simulink library "LopesDevelopmentLibrary"  (R2015b)
settings: Solver=ode45  StartTime=0.0  StopTime=10.0  RelTol=1e-3
values from neighbouring files (symbols this model uses):
  d2r = @(d) d*(pi/180)    [LopesDevelopmentLibrary_LoadParameters.m]
  ts = LopesParams.ts    [LopesDevelopmentLibrary_LoadParameters.m]
undefined symbols (not defined in the file or in its folder): anyParameterChanged, DiscIntNeverNeededParam, gcbh, LHF, LKF, LopesParams, macaddr, mxpcnetworkconfig, mxpcrtudprx, mxpcrtudptx, patientParametersChanged, port, PX, PZ, RHF, RKF, SelectorLOPESInSize, StrideTime_s, Time
undefined symbols (not defined in the file): LopesParamsSendDataArrayLen
libraries: LopesDevelopmentLibrary x288, simulink x98, dspmtrx3 x47, xpciplib x6, xpcnetworkbufferlib x5, dspsigops x4, dspstat3 x3, xpcethernetlib x2, visionstatistics x2, xpcseriallib x2, nmc x1, simulink_extras x1
(part 11 of 12)

== matlab function LopesDevelopmentLibrary/Robot control blocks/GeneralLopes/ShowStringInMatlabConsole1 ==
  data pre settings: description=Small string that is put in front of the received text.
  data: stringArray input; len input; pre input; enable input
function fcn(stringArray,len, pre, enable)
%#codegen
persistent t;
if isempty(t)
    t = 0;
end;
t = t+1;
    
coder.extrinsic('fprintf');
if (len~=0 && enable)
    fprintf('%6d: %s  (len = %d) - *%s*\n', t,char(pre'),len,char(stringArray(1:len).')); 
%    feval ('AddToGlobalXX',len);
end;

== matlab function LopesDevelopmentLibrary/Robot control blocks/FromLopes/ShowStringInMatlabConsole ==
  data pre settings: description=Small string that is put in front of the received text.
  data: stringArray input; len input; pre input; enable input
function fcn(stringArray,len, pre, enable)
%#codegen
persistent t;
if isempty(t)
    t = 0;
end;
t = t+1;
    
coder.extrinsic('fprintf');
if (len~=0 && enable)
    fprintf('%6d: %s  (len = %d) - *%s*\n', t,char(pre'),len,char(stringArray(1:len).')); 
%    feval ('AddToGlobalXX',len);
end;

== matlab function LopesDevelopmentLibrary/Robot control blocks/ToLopes/GenerateVelocities/MATLAB Function ==
  data: signalWidth input; forceType input; ena output
function ena = fcn(signalWidth,forceType)
%#codegen
ena=[0,0,0,0]; % We have four outputs
if forceType==-1
    if signalWidth==8
        ena(1)=1;
    else
        ena(2)=1;
    end;
else
    ena(forceType)=1;
end;

== matlab function LopesDevelopmentLibrary/StringFunctions/Pad/pad ==
  data: s input uint8; outArrayLen parameter; y output uint8; y_len output
function [y,y_len]= pad(s,outArrayLen)
%#codegen

% Given s, being an any-(fixed!)-length uint8-array, it outputs
% a 'string' array consisting of a default size (outArrayLen, as a
% parameter),padded with zero's
% together with a length indicating the number of 'valid' bytes in the
% string.
%
% If the string s is too long, it will use the first outputLen-1 chars (and
% add a null-char to fill the whole string up).

y = uint8(zeros(1,outArrayLen));
y_len = min(length(s), outArrayLen-1);
for i=1:y_len,
    y(i) = s(i);
end;

== matlab function LopesDevelopmentLibrary/Robot control blocks/ToLopes/ShowStringInMatlabConsoleIfNotEmpty2 ==
  data pre settings: description=Small string that is put in front of the received text.
  data: stringArray input; len input; pre input; enable input
function fcn(stringArray,len, pre, enable)
%#codegen
persistent t;
if isempty(t)
    t = 0;
end;
t = t+1;
    
coder.extrinsic('fprintf');
if (len~=0 && enable)
    fprintf('%6d: %s  (len = %d) - *%s*\n', t,char(pre'),len,char(stringArray(1:len).')); 
%    feval ('AddToGlobalXX',len);
end;

== matlab function LopesDevelopmentLibrary/StringFunctions/concatWithOptionalDelimiter ==
  data: s1 input; s1_len input; y output uint8; s2 input; s2_len input; y_len output; outputArrayLength parameter
function [y,y_len]= concatWithOptionalDelimiter(s1,s1_len, s2, s2_len, outputArrayLength)
%#codegen

% Concatenates s1 and s2 into y, using a specified delimiter if both strings are non-empty.
%
% s1 and s2 should be uint8-arrays containing a (possibly null-terminated) string.
% Usually, they will be a fixed-length array, holding the string in the
% first part; padded with zeros.
% s1_len and s2_len should be the actual string length (thus, the array
% uint8(['h','o','i',0,0,0,0]) has length 3. Use the strlen block for
% this.
%
% The result of this function is a fixed-length uint8-array, holding the
% string in the first part, padded with zeros, and the length of the
% resulting string (trailing zeros are not counted)
%
% If the resulting string would be too large to fit in the output array,
% it is truncated such that the output array is null-terminated and has
% maximum length.
%
% If s1_len> length(s1) (or similar with s2), the full length of the array
% will be taken as string.
%
% Note on outputArrayLength: The maximum string length is one less because of the trailing null-char

%% Parameters
delimiter = uint8(';'); % Examples: uint8(';'), uint8('; ')
                        % Cannot be a non-empty string (if you don't want a delimiter, remove it from the Add() lines.


%% The work itself

i = 1; % index within y
delimiter_len = length(delimiter);
y=uint8(zeros(outputArrayLength,1));

[y,i] = Add(s1, s1_len,              y, i, outputArrayLength);
if (s1_len~=0 && s2_len ~=0)
    [y,i] = Add(delimiter,delimiter_len, y, i, outputArrayLength);
end;
[y,i] = Add(s2, s2_len,              y, i, outputArrayLength);

y_len = i-1;

%-------------------------------------------------
%% This subfunction actually adds the given string. If the output string
% is alrady 'full', nothing happens.
function [y, i] = Add(whichArray, stringLength, y, i, outputArrayLength)
nToCopy = min([length(whichArray),stringLength, outputArrayLength - i]);
if (nToCopy~=0),
    y(i:(i+nToCopy-1)) = whichArray(1:nToCopy);
    i = i + nToCopy;
end;

== matlab function LopesDevelopmentLibrary/Robot control blocks/ToLopes/ShowStringInMatlabConsoleIfNotEmpty3 ==
  data pre settings: description=Small string that is put in front of the received text.
  data: stringArray input; len input; pre input; enable input
function fcn(stringArray,len, pre, enable)
%#codegen
persistent t;
if isempty(t)
    t = 0;
end;
t = t+1;
    
coder.extrinsic('fprintf');
if (len~=0 && enable)
    fprintf('%6d: %s  (len = %d) - *%s*\n', t,char(pre'),len,char(stringArray(1:len).')); 
%    feval ('AddToGlobalXX',len);
end;

== matlab function LopesDevelopmentLibrary/Robot control blocks/FromLopes/ShowStringInMatlabConsole1 ==
  data pre settings: description=Small string that is put in front of the received text.
  data: stringArray input; len input; pre input; enable input
function fcn(stringArray,len, pre, enable)
%#codegen
persistent t;
if isempty(t)
    t = 0;
end;
t = t+1;
    
coder.extrinsic('fprintf');
if (len~=0 && enable)
    fprintf('%6d: %s  (len = %d) - *%s*\n', t,char(pre'),len,char(stringArray(1:len).')); 
%    feval ('AddToGlobalXX',len);
end;

== matlab function LopesDevelopmentLibrary/StringFunctions/ShowStringInMatlabConsoleIfNotEmpty ==
  data pre settings: description=Small string that is put in front of the received text.
  data: stringArray input; len input; pre input; enable input
function fcn(stringArray,len, pre, enable)
%#codegen
persistent t;
if isempty(t)
    t = 0;
end;
t = t+1;
    
coder.extrinsic('fprintf');
if (len~=0 && enable)
    fprintf('%6d: %s  (len = %d) - *%s*\n', t,char(pre'),len,char(stringArray(1:len).')); 
%    feval ('AddToGlobalXX',len);
end;

== matlab function LopesDevelopmentLibrary/Robot control blocks/ToLopes/makeCreateBiasForceSpring ==
  data: normalBool input; bool output boolean; forceBool input double
function bool  = makeBool(normalBool, forceBool)
%#codegen

% Passes normalBool if forceBool is -1; otherwise it forces the output
% to be equal to forceBool. In diagram:
%
% forceBool | normalBool || Output
% --------------------------------
%     -1    |   false    || false
%     -1    |   true     || true
%      0    |  dont'care || false
% otherwise |  dont'care || true

if forceBool==-1
    bool = normalBool;
elseif forceBool == 0
    bool = false;
else
    bool = true;
end;

== matlab function LopesDevelopmentLibrary/BlocksForInternalUse/GaitGeneration/OrderKeyEvents/SortKeyEvents ==
  data: kE input; kE_out output; Error output double; jointNumber input double
function [kE_out, Error]= fcn(kE, jointNumber)
%#codegen
%
% This function does two things:
% (0.) It does keyEventPhases mod 100 (so that they're in the range [0,100).
% 1. It checks whether the key events (after wrapping around 100) are
%    strictly increasing. If not, it generates an Exception.
%    Note that it is allowed that the key event with the lowest phase
%    is somewhere in the middle, e.g. [50, 66, 95, 101, 7, 20]' as the
%    first column is valid.
% 2. It sorts the key events such that they are strictly increasing (if
%    there are two key events at the same place, the 'first' is decreased a
%    tiny little bit (1e-10) in order to make sure they are strictly
%    increasing again. This whole step is always done, even if an exception
%    was generated.
%
% The underlying reasons:
% 1. If the key events are not in the right order, this is most probably not
%    what we want, so we should stop the whole thing.
% 2. The blocks further on in the data path require a strictly incrasing
%    key event matrix. In order to guarantee that these blocks don't crash,
%    we will make sure that they get what they want, even if the resulting
%    data would not be what we want. The exception can be used to detect
%    this situation, and at least the application does not crash.
%
% Example:
%      [  50   101   102   103 ]
%      [  66   201   202   203 ] 
%      [  95   301   302   303 ]
%  In: [ 101   401   402   403 ]
%      [   7   501   502   503 ]
%      [  20   601   602   603 ]
%  

% Get phase data and wrap them
firstColumn = mod(kE(:,1),100);
kE (:,1) = firstColumn;

% Strict increasingness can be checked by getting the diff of the phase
% data; there should be only one value <=0
nNonPositives = sum(diff([firstColumn;firstColumn(1)]) <=0);

% Exception handling
if (nNonPositives~=1),
    % Then the key events are not in correct order
    Error=jointNumber;
else
    % No error
    Error=0;
end;

while true
    % Sort them (no guarantee on identicity of two adjacent key events
    kE = sortrows(kE,1);

    % Check if we have multiple key events at one spot
    firstColumn = kE(:,1);
    d = diff(firstColumn);
    if (all(d~=0)), break; end; % Then there are no overlaps
    firstColumn(d==0) = mod(firstColumn(d==0)-1,100);
    kE(:,1) = firstColumn;
end;

kE_out = kE;

== matlab function LopesDevelopmentLibrary/BlocksForInternalUse/GaitGeneration/keyEvents2breakscoefs3/keyEvents2breakscoefs3 ==
  data: keyEvents input; breaks output; coefs output
function [breaks,coefs] = keyEvents2breakscoefs3(keyEvents)
%#codegen
%
% Given key-events with x, position and velocity, this function creates
% breaks/coefs for a 3rd order spline

% This function generates a list of breaks and coefs, given a list
% of keyEvents. The keyEvents matrix should have one row for each 'event',
% being [time, position, rate].
% Units:
% - phase [%]
% - position [deg, cm, ...]
% - rate [deg/%, cm/%, ...]
%
% The values in phase should be strictly increasing and 0<=phase<100.
% This function automatically wraps the events, so there is no need to put
% an event at 0.

% Add a key event before zero and one after 100:
kE = [ ...
    keyEvents(end,:) - [100,0,0];
    keyEvents;
    keyEvents(1,:) + [100,0,0]];

% Special case: it may be the case that the user gave a key event at exactly 0 AND
% at exactly 100. In that case, we get repeated key events at 0 and 100
% (because of the previous operation), which is invalid for ppval. We can
% not throw the extra points away because the length of the array is fixed.
% However, we can move them away freely because we will never use the parts
% below 0 and above 100 (and the part between 0 and 100 is not affected).
% Note however that this may give a jump in the position (or velocity)
% of the signal. Therefore, this actually should never happen (with the
% exception of the time signal).
if (kE(1,1) == 0 && kE(2,1) == 0)
    kE(1,1) = -100;
    kE(end,1) = 200;
end;
% For the generation of piecewise polynomials, we need the endpoint data
% of two breaks in one line, so build a matrix:
kE2 = [kE(1:end-1,2:3), kE(2:end,2:3)];

breaks = kE(:,1);
diffbreaks = diff(breaks);
coefs=zeros(size(kE2,1),4); 
for i=1:size(kE2,1),
    % x1 = 0;
    x2 = diffbreaks(i);

    % In theory:
    %   A = [  x1^3,   x1^2,   x1,   1; 
    %        3*x1^2, 2*x1  ,    1,   0;
    %          x2^3,   x2^2,   x2,   1;
    %        3*x2^2, 2*x2  ,    1,   0];
    % However, x1=0, so it becomes:
    A = [0, 0, 0, 1; 0, 0, 1,0; x2^3, x2^2, x2, 1; 3*x2^2, 2*x2, 1,0]; 
    coefs(i,:) = (A \ (kE2(i,:))')';
end;

% pp = mkpp(breaks,coefs);

== matlab function LopesDevelopmentLibrary/StringFunctions/concatDelimiter ==
  data: s1 input; s1_len input; y output; s2 input; s2_len input; y_len output
function [y,y_len]= concatDelimiter(s1,s1_len, s2, s2_len)
%#codegen

% Concatenates s1 and s2 into y, using a ';' as a delimiter.
%
% s1 and s2 should be uint8-arrays containing a (possibly null-terminated) string.
% Usually, they will be a fixed-length array, holding the string in the
% first part; padded with zeros.
% s1_len and s2_len should be the actual string length (thus, the array
% uint8(['h','o','i',0,0,0,0]) has length 3. Use the strlen block for
% this.
%
% The result of this function is a fixed-length uint8-array, holding the
% string in the first part, padded with zeros, and the length of the
% resulting string (trailing zeros are not counted)
%
% If the resulting string would be too large to fit in the output array,
% it is truncated such that the output array is null-terminated and has
% maximum length.
%
% If s1_len> length(s1) (or similar with s2), the full length of the array
% will be taken as string.

%% Parameters
outputArrayLength = uint32(100); % The maximum string length is one less because of the trailing null-char
delimiter = uint8(';'); % Examples: uint8(';'), uint8('; ')
                        % Cannot be a non-empty string (if you don't want a delimiter, remove it from the Add() lines.
delimiter_len = 1;


%% The work itself
i = uint32(1); % index within y
y=zeros(outputArrayLength,1);

[y,i] = Add(s1, s1_len,              y, i, outputArrayLength);
[y,i] = Add(delimiter,delimiter_len, y, i, outputArrayLength);
[y,i] = Add(s2, s2_len,              y, i, outputArrayLength);

y_len = i-1;

%-------------------------------------------------
%% This subfunction actually adds the given string. If the output string
% is alrady 'full', nothing happens.
function [y, i] = Add(whichArray, stringLength, y, i, outputArrayLength)
nToCopy = min([length(whichArray),stringLength, outputArrayLength - i]);
if (nToCopy~=0),
    y(i:(i+nToCopy-1)) = whichArray(1:nToCopy);
    i = i + nToCopy;
end;

== matlab function LopesDevelopmentLibrary/StringFunctions/strlen_as_double ==
  data: s input; len output
function len = strlen(s)
%#codegen

% This function returns the length of the actual string, WITHOUT any
% trailing '\0's. So, the array  ['h','e','l','l','o',0,0,0,0] returns 5.0.
% The output of this function is a double.
%
% s should be a uint8-array containing a string terminated with at least
% one '\0' character. The ASCII Encode block generates such an array
% (the array generated is fixed length, the first n bytes are the string,
% all other bytes are '\0'). 
%
% If the string does not have a trailing '\0' (in other words, if it is
% too large for its containing array), it returns the length of the array.

len = 1.0;
maxlen = length(s);

while (len<= maxlen && s(len)~=0), 
    len = len + 1; 
end;
% Now len is the index of the first trailing '\0' (or maxlen+1);
% that is one more than the string length, so decrease by one:
len = len - 1;

== matlab function LopesDevelopmentLibrary/BlocksForInternalUse/GaitGeneration/keyEvents2breakscoefs5/keyEvents2breakscoefs5 ==
  data: keyEvents input; breaks output; coefs output
function [breaks,coefs] = keyEvents2breakscoefs5(keyEvents)
%#codegen
%
% Given key-events with x, position, velocity and acceleration, this
% function creates breaks/coefs for a 5rd order spline

% This function generates a list of breaks and coefs, given a list
% of keyEvents. The keyEvents matrix should have one row for each 'event',
% being [time, position, rate, rate^2].
% Units:
% - phase [%]
% - position [rad, m, ...]
% - rate [rad/%, m/%, ...]
% - rate^2 [ rad/%^2, m/%^2, ...]
%
% The values in phase should be strictly increasing and 0<=phase<100.
% This function automatically wraps the events, so there is no need to put
% an event at 0.

% Add a key event before zero and one after 100:
kE = [ ...
    keyEvents(end,:) - [100,0,0,0];
    keyEvents;
    keyEvents(1,:) + [100,0,0,0]];

% Special case: it may be the case that the user gave a key event at exactly 0 AND
% at exactly 100. In that case, we get repeated key events at 0 and 100
% (because of the previous operation), which is invalid for ppval. We can
% not throw the extra points away because the length of the array is fixed.
% However, we can move them away freely because we will never use the parts
% below 0 and above 100 (and the part between 0 and 100 is not affected).
% Note however that this may give a jump in the position (or velocity)
% of the signal. Therefore, this actually should never happen (with the
% exception of the time signal).
if (kE(1,1) == 0 && kE(2,1) == 0)
    kE(1,1) = -100;
    kE(end,1) = 200;
end;
% For the generation of piecewise polynomials, we need the endpoint data
% of two breaks in one line, so build a matrix:
kE2 = [kE(1:end-1,2:4), kE(2:end,2:4)];

breaks = kE(:,1);
diffbreaks = diff(breaks);
coefs=zeros(size(kE2,1),6); 
for i=1:size(kE2,1),
    % x1 = 0;
    x2 = diffbreaks(i);

    % In theory:
    % y1   = coefs1 *    x1^5 + coefs2 *    x1^4 + ...
    % y1'  = coefs1 *  5*x1^4 + coefs2 *  4*x1^3 + ...
    % y1'' = coefs1 * 20*x1^3 + coefs2 * 12*x1^2 + ...
    %
    % thus: Y = A * C with:
    %
    %     [ y1   ]      [    x1^5      x1^4     x1^3    x1^2  x1  1 ]     [ coefs1 ]
    %     [ y1'  ]      [  5*x1^4    4*x1^3   3*x1^2  2*x1    1   0 ]     [ coefs2 ]
    % Y=  [ y1'' ]  A = [ 20*x1^3   12*x1^2   6*x1       2    0   0 ] C = [ coefs3 ]
    %     [ y2   ]      [    x2^5      x2^4     x2^3    x2^2  x2  1 ]     [ coefs4 ]
    %     [ y2'  ]      [  5*x2^4    4*x2^3   3*x2^2  2*x2    1   0 ]     [ coefs5 ]
    %     [ y2'' ]      [ 20*x2^3   12*x2^2   6*x2       2    0   0 ]     [ coefs6 ]
    x2_2 = x2  *x2; % Powers of x2; precalculate because we need them often
    x2_3 = x2_2*x2;
    x2_4 = x2_2*x2_2;
    x2_5 = x2_3*x2_2;
    % However, x1=0, so it becomes:
    A = [   0        0       0       0      0     1;
            0        0       0       0      1     0;
            0        0       0       2      0     0;
           x2_5,    x2_4,   x2_3,   x2_2,  x2,    1;
         5*x2_4,  4*x2_3, 3*x2_2, 2*x2,     1,    0;
        20*x2_3, 12*x2_2, 6*x2,      2,     0,    0 ];
    coefs(i,:) = (A \ (kE2(i,:))')';
end;

% pp = mkpp(breaks,coefs);

== matlab function LopesDevelopmentLibrary/StringFunctions/concat5/concat5 ==
  data: s1 input; s1_len input; y output size=outStrLen; s2 input; s2_len input; y_len output; s3 input; s3_len input; s4 input; s4_len input; s5 input; s5_len input size=1; outStrLen parameter
function [y,y_len]= concat5(s1,s1_len, s2, s2_len,s3,s3_len, s4, s4_len, s5, s5_len, outStrLen)
%#codegen

% Concatenates s1 and s2, ... into y, using a specified delimiter.
%
% s1 and s2 should be uint8-arrays containing a (possibly null-terminated) string.
% Usually, they will be a fixed-length array, holding the string in the
% first part; padded with zeros.
% s1_len and s2_len should be the actual string length (thus, the array
% uint8(['h','o','i',0,0,0,0]) has length 3. Use the strlen block for
% this.
%
% The result of this function is a fixed-length uint8-array, holding the
% string in the first part, padded with zeros, and the length of the
% resulting string (trailing zeros are not counted)
%
% If the resulting string would be too large to fit in the output array,
% it is truncated such that the output array is null-terminated and has
% maximum length.
%
% If s1_len> length(s1) (or similar with s2), the full length of the array
% will be taken as string.

%% Parameters
outputArrayLength = uint32(outStrLen); % The maximum string length is one less because of the trailing null-char


%% The work itself

i =uint32(1); % index within y
y=uint8(zeros(outputArrayLength,1));

[y,i] = Add(s1, s1_len, y, i, outputArrayLength);
[y,i] = Add(s2, s2_len, y, i, outputArrayLength);
[y,i] = Add(s3, s3_len, y, i, outputArrayLength);
[y,i] = Add(s4, s4_len, y, i, outputArrayLength);
[y,i] = Add(s5, s5_len, y, i, outputArrayLength);

y_len = double(i-1);

%-------------------------------------------------
%% This subfunction actually adds the given string. If the output string
% is alrady 'full', nothing happens.
function [y, i] = Add(whichArray, stringLength, y, i, outputArrayLength)
nToCopy = min([length(whichArray),stringLength, outputArrayLength - i]);
if (nToCopy~=0),
    y(i:(i+nToCopy-1)) = whichArray(1:nToCopy);
    i = i + nToCopy;
end;

== matlab function LopesDevelopmentLibrary/BlocksForInternalUse/GaitGeneration/RegressionData2KeyEvents/RegressionData2KeyEvents ==
  data: regressionParameters input; keyEvents output; v input; bodyLength input
function keyEvents = RegressionData2KeyEvents(regressionParameters, v, bodyLength)
%#codegen
%
% This function generates a list of key events from regression parameters.
%
% Format keyEvents:
% - One key event per row
% - For each row (i.e., each key event):
%   [x, y, dydx] or [x, y, dydx, ddydx] (depending on the size of regressionparameters)
%   The units are the same as the units of the regressionParameters (they are:
%   v [m/s]; l [m]; phase [%]; joint angle [rad]; joint ang.vel [rad/%]; joint ang.acc [rad/%^2])
%
% Format regressionparameters:
% - One key event per row
% - For each row (i.e., each key event):
%   + First  four elements  (1:4) are regression parameters for first element in keyEvents (i.e., x),
%   + Second four elements  (5:8) are regression parameters for second element in keyEvents (i.e., y)
%   + Third  four elements (9:12) are regression parameters for third element in keyEvents (i.e., dydx)
%   + Fourth four elements (13:16) (if they exist) are regression parameters for fourth element in keyEvents (i.e., ddydx)
%
% In order to get the key Event parameters from the regression parameters,
% we apply the following formula:
%
%      key = reg1 + reg2 * v + reg3 * v^2 + reg4 * l
%
% where:
%   - key is the resulting keyEvent parameter
%   - reg1..4 are the regression parameters
%   - v is the walking velocity in m/s
%
% You can obtain this from Bram's data by, using the GenerateGaitDataBramVariable.m script.

% Make sure we have a column vector
if size(regressionParameters,2) == 1
    regressionParametersFlip = regressionParameters';
else
    regressionParametersFlip = regressionParameters;
end

keyEvents = zeros(size(regressionParametersFlip)./[1,4]);

y = [1; v; v^2; bodyLength];
for i = 1: size(keyEvents,2),
    ii = (i*4-3):(i*4);
    keyEvents(:,i) = regressionParametersFlip (:,ii) * y;
end;

== matlab function LopesDevelopmentLibrary/BlocksForInternalUse/LLC Communication/LLCSendUDP/ShowInMatlabConsole IfNotEmpty ==
  data pre settings: description=Small string that is put in front of the received text.
  data: stringArray input; len input; pre input; enable input
function fcn(stringArray,len, pre, enable)
%#codegen
persistent t;
if isempty(t)
    t = 0;
end;
t = t+1;
    
coder.extrinsic('fprintf');
if (len~=0 && enable)
    fprintf('%6d: %s  (len = %d) - *%s*\n', t,char(pre'),len,char(stringArray(1:len).')); 
%    feval ('AddToGlobalXX',len);
end;

== matlab function LopesDevelopmentLibrary/BlocksForInternalUse/LLC Communication/LLCReceiveUDP/ShowInMatlabConsoleIfNotEmpty ==
  data pre settings: description=Small string that is put in front of the received text.
  data: stringArray input; len input; pre input; enable input
function fcn(stringArray,len, pre, enable)
%#codegen
persistent t;
if isempty(t)
    t = 0;
end;
t = t+1;
    
coder.extrinsic('fprintf');
if (len~=0 && enable)
    fprintf('%6d: %s  (len = %d) - *%s*\n', t,char(pre'),len,char(stringArray(1:len).')); 
%    feval ('AddToGlobalXX',len);
end;

== matlab function LopesDevelopmentLibrary/BlocksForInternalUse/GaitGeneration/CalculateReferenceGait/CalculateAbductionLeft/MATLAB Function ==
  data: isRight input; Abduction output; PelvisTZ input; dPelvisTZdx input; ddPelvisTZdx input; AnkleTZ input; dAnkleTZdx input; ddAnkleTZdx input; xHF input; dxHFdx input; ddxHFdx input; xKF input; dxKFdx input; ddxKFdx input; w_pelvis input; l_upper input; l_lower input; dAbductiondx output; ddAbductiondx output
function [Abduction,dAbductiondx,ddAbductiondx]= fcn(isRight,PelvisTZ,dPelvisTZdx,ddPelvisTZdx, ...
    AnkleTZ,dAnkleTZdx,ddAnkleTZdx, ...
    xHF, dxHFdx, ddxHFdx, xKF, dxKFdx, ddxKFdx,...
    w_pelvis, l_upper, l_lower ) % Constants
%#codegen
%
% Given the above parameters, it calculates the abduction needed to
% (approximately) get the sideways position of the ankle (AnkleTZ) to the
% given value. We could do the analytical derivative, but that's a nasty
% function, so let's try with numerical derivative first...

% Explanation:
%
% We can express the sideways position of the ankle (of any foot) as:
%
% AnkleTZ = PelvisTZ + U * 0.5 * wPelvis + U * sin(xHA) * l_leg_projected
%
% with U = 1 for Right leg; U = -1 for left leg.
%      l_leg_projected is the length of the leg, projected onto
%            the yz plane: l_leg_projected = cos(xHF) * l_upper + cos(xHF-xKF) * l_lower
%      wPelvis is the distance between the hip rotation points (approx 0.2 m)
%
% Note that this equation ignores any pelvis rotations.
%
% Solving for xHA, we get (note that U^2=1 always):
%             /     U (AnkleTZ-PelvisTZ) - 0.5* wPelvis     \
% xHA = asin |  -------------------------------------------  |
%             \ cos(xHF) * l_upper + cos(xHF-xKF) * l_lower /
% 
% We could get the analytical derivative, but that's nasty to find. So,
% let's first go for the numerical derivative

% Original code; now obsolete because I also calculate analytical
% derivatives and I need parts of the equation for it:
%  if (isRight), U=1; else U=-1; end;
%  l_leg_projected = cos(xHF) * l_upper + cos(xHF-xKF) * l_lower;
%  Abduction = asin ( (U* (AnkleTZ - PelvisTZ) - (0.5*wPelvis)) / l_leg_projected);

% In order to get the derivatives also, we split up the equation into
% xHA = asin ( T / N ), with T = U(ATZ-PTZ)-0.5wPelvis; N = l_leg_projected
if (isRight), U=1; else U=-1; end;
T = U* (AnkleTZ - PelvisTZ) - 0.5*w_pelvis;
dTdx = U * (dAnkleTZdx - dPelvisTZdx);
ddTdx = U * (ddAnkleTZdx - ddPelvisTZdx);

N = cos(xHF) * l_upper + cos(xHF-xKF) * l_lower;
dNdx = -l_upper * sin(xHF) * dxHFdx - l_lower * sin(xHF-xKF) * (dxHFdx - dxKFdx);
ddNdx = -l_upper * (cos(xHF) * dxHFdx^2 + sin(xHF) * ddxHFdx) - l_lower * (cos(xHF-xKF)* (dxHFdx-dxKFdx)^2 + sin(xHF-xKF) * (ddxHFdx - ddxKFdx));

TN = T/N;
dTNdx = dTdx / N -  (T/(N^2)) * dNdx;
ddTNdx = ddTdx/N - dTdx/N^2*dNdx   -   dTdx/N^2*dNdx + T*dNdx * 2 * N^-3 * dNdx - T/N^2 * ddNdx;

Abduction = asin ( T/N);
dAbductiondx = dTNdx/sqrt(1-TN^2); % = dTNdx * (1-TN^2)^(-1/2)
ddAbductiondx = ddTNdx/sqrt(1-TN^2) + dTNdx * ( -(1/2) * (1-TN^2)^(-3/2) * -2*TN * dTNdx);

return;

% %% Code to prove the equations are right:
% syms PelvisTZ(t) AnkleTZ(t) xHF(t) xKF(t)
% syms l_upper l_lower w_pelvis U
% ss0 = {'PelvisTZ(t)','AnkleTZ(t)','xHF(t)','xKF(t)'};
% sr0 = {'PelvisTZ','AnkleTZ','xHF','xKF'};
% ss1 = {'D(PelvisTZ)(t)','D(AnkleTZ)(t)','D(xHF)(t)','D(xKF)(t)'};
% sr1 = {'dPelvisTZdx','dAnkleTZdx','dxHFdx','dxKFdx'};
% ss2 = {'D(D(PelvisTZ))(t)','D(D(AnkleTZ))(t)','D(D(xHF))(t)','D(D(xKF))(t)'};
% sr2 = {'ddPelvisTZdx','ddAnkleTZdx','ddxHFdx','ddxKFdx'};
% ss = {ss2{:}, ss1{:}, ss0{:}};
% sr = {sr2{:}, sr1{:}, sr0{:}};
% 
% 
% l_leg_projected = cos(xHF) * l_upper + cos(xHF-xKF) * l_lower;
% Ab2 = asin ( (U* (AnkleTZ - PelvisTZ) - (0.5*w_pelvis)) / l_leg_projected);
% dAb2= simple(diff(Ab2,t));
% ddAb2 = diff(dAb2,t);
% 
% Ab3 = subs(Ab2,ss,sr)
% dAb3 = subs(dAb2,ss,sr) % This is the derivative according to matlab
% ddAb3 = subs(ddAb2,ss,sr) % This is the second derivative according to matlab
% 
% % Copy my own equations as syms
% syms PelvisTZ dPelvisTZdx ddPelvisTZdx  ...
%     AnkleTZ dAnkleTZdx ddAnkleTZdx  ...
%     xHF  dxHFdx  ddxHFdx xKF dxKFdx ddxKFdx...
%     w_pelvis l_upper l_lower
% 
% T = U* (AnkleTZ - PelvisTZ) - 0.5*w_pelvis;
% dTdx = U * (dAnkleTZdx - dPelvisTZdx);
% ddTdx = U * (ddAnkleTZdx - ddPelvisTZdx);
% 
% N = cos(xHF) * l_upper + cos(xHF-xKF) * l_lower;
% dNdx = -l_upper * sin(xHF) * dxHFdx - l_lower * sin(xHF-xKF) * (dxHFdx - dxKFdx);
% ddNdx = -l_upper * (cos(xHF) * dxHFdx^2 + sin(xHF) * ddxHFdx) - l_lower * (cos(xHF-xKF)* (dxHFdx-dxKFdx)^2 + sin(xHF-xKF) * (ddxHFdx - ddxKFdx));
% 
% TN = T/N;
% dTNdx = dTdx / N -  (T/(N^2)) * dNdx;
% %ddTNdx = ddTdx/N - dTdx/N^2 * dNdx  - (dTdx/N^2 - 2*T/N^3 * dNdx + (T/N^2)*ddNdx);
% ddTNdx = ddTdx/N - dTdx/N^2*dNdx   -   dTdx/N^2*dNdx + T*dNdx * 2 * N^-3 * dNdx - T/N^2*ddNdx;
% 
% Abduction = asin ( T/N)
% dAbductiondx = simple(dTNdx/sqrt(1-TN^2)) % = dTNdx * (1-TN^2)^(-1/2)
% ddAbductiondx = ddTNdx/sqrt(1-TN^2) + dTNdx * ( -(1/2) * (1-TN^2)^(-3/2) * -2*TN * dTNdx)
% 
% % Check if they're the same; these should all be zero
% er0 = simple(Ab3 - Abduction)
% er1 = simple(dAbductiondx - dAb3)
% er2 = ddAbductiondx - ddAb3
% 
% % er2 is too complex to show analytically. Therefore, let's use random
% %% numbers to show
% U=1;
% PelvisTZ=rand/5; dPelvisTZdx=rand; ddPelvisTZdx=rand;
% AnkleTZ=rand/5; dAnkleTZdx=rand;ddAnkleTZdx=rand;
% xHF=rand/5; dxHFdx=rand; ddxHFdx=rand; xKF=rand/2; dxKFdx=rand; ddxKFdx=rand;
% w_pelvis=abs(rand); l_upper=abs(rand); l_lower=abs(rand);
% (((w_pelvis/2 - U*(AnkleTZ - PelvisTZ))*(ddxHFdx*l_upper*sin(xHF) + dxHFdx^2*l_upper*cos(xHF) + l_lower*sin(xHF - xKF)*(ddxHFdx - ddxKFdx) + l_lower*cos(xHF - xKF)*(dxHFdx - dxKFdx)^2))/(l_upper*cos(xHF) + l_lower*cos(xHF - xKF))^2 + (2*(w_pelvis/2 - U*(AnkleTZ - PelvisTZ))*(dxHFdx*l_upper*sin(xHF) + l_lower*sin(xHF - xKF)*(dxHFdx - dxKFdx))^2)/(l_upper*cos(xHF) + l_lower*cos(xHF - xKF))^3 - (U*(ddAnkleTZdx - ddPelvisTZdx))/(l_upper*cos(xHF) + l_lower*cos(xHF - xKF)) - (2*U*(dAnkleTZdx - dPelvisTZdx)*(dxHFdx*l_upper*sin(xHF) + l_lower*sin(xHF - xKF)*(dxHFdx - dxKFdx)))/(l_upper*cos(xHF) + l_lower*cos(xHF - xKF))^2)/(1 - (w_pelvis/2 - U*(AnkleTZ - PelvisTZ))^2/(l_upper*cos(xHF) + l_lower*cos(xHF - xKF))^2)^(1/2) - ((2*(w_pelvis/2 - U*(AnkleTZ - PelvisTZ))*(dxHFdx*l_upper*sin(xHF) + l_lower*sin(xHF - xKF)*(dxHFdx - dxKFdx))^2)/(l_upper*cos(xHF) + l_lower*cos(xHF - xKF))^3 - (U*(ddAnkleTZdx - ddPelvisTZdx))/(l_upper*cos(xHF) + l_lower*cos(xHF - xKF)) + ((w_pelvis/2 - U*(AnkleTZ - PelvisTZ))*(l_lower*(sin(xHF - xKF)*(ddxHFdx - ddxKFdx) + cos(xHF - xKF)*(dxHFdx - dxKFdx)^2) + l_upper*(cos(xHF)*dxHFdx^2 + ddxHFdx*sin(xHF))))/(l_upper*cos(xHF) + l_lower*cos(xHF - xKF))^2 - (2*U*(dAnkleTZdx - dPelvisTZdx)*(dxHFdx*l_upper*sin(xHF) + l_lower*sin(xHF - xKF)*(dxHFdx - dxKFdx)))/(l_upper*cos(xHF) + l_lower*cos(xHF - xKF))^2)/(1 - (w_pelvis/2 - U*(AnkleTZ - PelvisTZ))^2/(l_upper*cos(xHF) + l_lower*cos(xHF - xKF))^2)^(1/2) - (((2*(w_pelvis/2 - U*(AnkleTZ - PelvisTZ))^2*(dxHFdx*l_upper*sin(xHF) + l_lower*sin(xHF - xKF)*(dxHFdx - dxKFdx)))/(l_upper*cos(xHF) + l_lower*cos(xHF - xKF))^3 - (2*U*(w_pelvis/2 - U*(AnkleTZ - PelvisTZ))*(dAnkleTZdx - dPelvisTZdx))/(l_upper*cos(xHF) + l_lower*cos(xHF - xKF))^2)*((U*(dAnkleTZdx - dPelvisTZdx))/(l_upper*cos(xHF) + l_lower*cos(xHF - xKF)) - ((w_pelvis/2 - U*(AnkleTZ - PelvisTZ))*(dxHFdx*l_upper*sin(xHF) + l_lower*sin(xHF - xKF)*(dxHFdx - dxKFdx)))/(l_upper*cos(xHF) + l_lower*cos(xHF - xKF))^2))/(2*(1 - (w_pelvis/2 - U*(AnkleTZ - PelvisTZ))^2/(l_upper*cos(xHF) + l_lower*cos(xHF - xKF))^2)^(3/2)) - ((w_pelvis/2 - U*(AnkleTZ - PelvisTZ))*((U*(dAnkleTZdx - dPelvisTZdx))/(l_upper*cos(xHF) + l_lower*cos(xHF - xKF)) - ((w_pelvis/2 - U*(AnkleTZ - PelvisTZ))*(dxHFdx*l_upper*sin(xHF) + l_lower*sin(xHF - xKF)*(dxHFdx - dxKFdx)))/(l_upper*cos(xHF) + l_lower*cos(xHF - xKF))^2)^2)/((1 - (w_pelvis/2 - U*(AnkleTZ - PelvisTZ))^2/(l_upper*cos(xHF) + l_lower*cos(xHF - xKF))^2)^(3/2)*(l_upper*cos(xHF) + l_lower*cos(xHF - xKF)))
% % Indeed, it gives 0!

== matlab function LopesDevelopmentLibrary/BlocksForInternalUse/GaitGeneration/ppval_bus/ppval ==
  data: xx input; yy output; breaks input; coefs input; dydx output; ddydx output
function [yy, dydx,ddydx] = ppval(xx,breaks, coefs)
%#codegen

%% same functionality as ppval but without using structs as input. 

%  obtain the row vector xs equivalent to XX
lx = numel(xx); 
xs = reshape(xx,lx,1);

%get order of spline(k) and number of pieces(l)
[l,k]=size(coefs);

% for each element of xx, compute the breakpoint interval
[~,index] = histc(xs,[-inf;breaks(2:l);inf]);

% now go to local coordinates ...
xs = xs-breaks(index);

% ... and apply nested multiplication:
yy = coefs(index,1);
for i=2:k
   yy = xs(:).*yy + coefs(index,i);
end

dydx = coefs(index,1)*(k-1);
for i=2:k-1
   dydx = xs(:).*dydx + coefs(index,i)*(k-i);
end

ddydx = coefs(index,1)*(k-1)*(k-2);
for i=2:k-2
   ddydx = xs(:).*ddydx + coefs(index,i)*(k-i)*(k-i-1);
end

== matlab function LopesDevelopmentLibrary/BlocksForInternalUse/GaitGeneration/TrajectoryOfInfluence/TrajectoryOfInfluence ==
  data: parameters input; keyEventTimes input; phase input; alpha output
function alpha=TrajectoryOfInfluence(parameters, keyEventTimes, phase)
% Given all parameters, it returns the 'Trajectory of influence \in [0,1] according to this profile, at the current phase.
% For a detailed description, see the Technical Documentation.

startEventIndex = parameters(1);
startDuration   = parameters(2);
endEventIndex   = parameters(3);
endDuration     = parameters(4);

% Durations are not allowed to be 50 or more (so limit them to 49). They also should be strictly positive
if (startDuration>49), startDuration = 49; end;
if (endDuration>49), endDuration = 49; end;
if (startDuration <1), startDuration = 1; end;
if (endDuration < 1), endDuration = 1; end;


phi_start = keyEventTimes(startEventIndex);
phi_end   = keyEventTimes(endEventIndex);

% Calculate starting and ending point of ramps up and down
s1 = phi_start - startDuration/2;
s2 = phi_start + startDuration/2;
e1 = phi_end   - endDuration/2;
e2 = phi_end   + endDuration/2;

% Calculate the value of the ramp up and down at this specific phi
% (NaN if it is outside the ramp)
if withinRange(phase,s1,s2)
    U = wrap(phase - s1)/wrap(s2-s1);
else
    U = NaN;
end;

if withinRange(phase,e1,e2)
    D = wrap(e2-phase) / wrap(e2-e1);
else
    D = NaN;
end;

% There may be overlap between the ramps; depending on where the overlap
% can be, we need one of the two equations below. See also the Technical
% Documentation
if wrap(phi_end-phi_start)<=50,
    if withinRange(phase,s1,e2)
        alpha = min([U,D,1]);
    else
        alpha = 0;
    end;
else
    if withinRange(phase,e1,s2)
        alpha = max([U,D,0]);
    else
        alpha = 1;
    end;
end;
    

function Y = withinRange(x,minn,maxx)
% Returns true (1) if x is within the range [minn,maxx] (including these limits),
% while keeping wrapping in mind. Examples:
% withinRange (20,10,30) -> True
% withinRange (90,99,10) -> True
% withinRange (40,40,40) -> True
% withinRange (50,49,51) -> True
% withinRange (40,10,40) -> False
% withinRange (50,51,49) -> False
x = mod(x,100); minn = mod(minn,100); maxx=mod(maxx,100);
if (minn<=maxx && (minn<= x && x <=maxx)), Y=1;
elseif (minn>maxx && (minn<=x || x<=maxx)), Y=1;
else Y=0;
end;

function y = wrap(x)
% Returns x, wrapped to the range [0,100)
y = mod(x,100);

== matlab function LopesDevelopmentLibrary/BlocksForInternalUse/GaitGeneration/CalculateReferenceGait/CalculateAbductionRight/MATLAB Function ==
  data: isRight input; Abduction output; PelvisTZ input; dPelvisTZdx input; ddPelvisTZdx input; AnkleTZ input; dAnkleTZdx input; ddAnkleTZdx input; xHF input; dxHFdx input; ddxHFdx input; xKF input; dxKFdx input; ddxKFdx input; w_pelvis input; l_upper input; l_lower input; dAbductiondx output; ddAbductiondx output
function [Abduction,dAbductiondx,ddAbductiondx]= fcn(isRight,PelvisTZ,dPelvisTZdx,ddPelvisTZdx, ...
    AnkleTZ,dAnkleTZdx,ddAnkleTZdx, ...
    xHF, dxHFdx, ddxHFdx, xKF, dxKFdx, ddxKFdx,...
    w_pelvis, l_upper, l_lower ) % Constants
%#codegen
%
% Given the above parameters, it calculates the abduction needed to
% (approximately) get the sideways position of the ankle (AnkleTZ) to the
% given value. We could do the analytical derivative, but that's a nasty
% function, so let's try with numerical derivative first...

% Explanation:
%
% We can express the sideways position of the ankle (of any foot) as:
%
% AnkleTZ = PelvisTZ + U * 0.5 * wPelvis + U * sin(xHA) * l_leg_projected
%
% with U = 1 for Right leg; U = -1 for left leg.
%      l_leg_projected is the length of the leg, projected onto
%            the yz plane: l_leg_projected = cos(xHF) * l_upper + cos(xHF-xKF) * l_lower
%      wPelvis is the distance between the hip rotation points (approx 0.2 m)
%
% Note that this equation ignores any pelvis rotations.
%
% Solving for xHA, we get (note that U^2=1 always):
%             /     U (AnkleTZ-PelvisTZ) - 0.5* wPelvis     \
% xHA = asin |  -------------------------------------------  |
%             \ cos(xHF) * l_upper + cos(xHF-xKF) * l_lower /
% 
% We could get the analytical derivative, but that's nasty to find. So,
% let's first go for the numerical derivative

% Original code; now obsolete because I also calculate analytical
% derivatives and I need parts of the equation for it:
%  if (isRight), U=1; else U=-1; end;
%  l_leg_projected = cos(xHF) * l_upper + cos(xHF-xKF) * l_lower;
%  Abduction = asin ( (U* (AnkleTZ - PelvisTZ) - (0.5*wPelvis)) / l_leg_projected);

% In order to get the derivatives also, we split up the equation into
% xHA = asin ( T / N ), with T = U(ATZ-PTZ)-0.5wPelvis; N = l_leg_projected
if (isRight), U=1; else U=-1; end;
T = U* (AnkleTZ - PelvisTZ) - 0.5*w_pelvis;
dTdx = U * (dAnkleTZdx - dPelvisTZdx);
ddTdx = U * (ddAnkleTZdx - ddPelvisTZdx);

N = cos(xHF) * l_upper + cos(xHF-xKF) * l_lower;
dNdx = -l_upper * sin(xHF) * dxHFdx - l_lower * sin(xHF-xKF) * (dxHFdx - dxKFdx);
ddNdx = -l_upper * (cos(xHF) * dxHFdx^2 + sin(xHF) * ddxHFdx) - l_lower * (cos(xHF-xKF)* (dxHFdx-dxKFdx)^2 + sin(xHF-xKF) * (ddxHFdx - ddxKFdx));

TN = T/N;
dTNdx = dTdx / N -  (T/(N^2)) * dNdx;
ddTNdx = ddTdx/N - dTdx/N^2*dNdx   -   dTdx/N^2*dNdx + T*dNdx * 2 * N^-3 * dNdx - T/N^2 * ddNdx;

Abduction = asin ( T/N);
dAbductiondx = dTNdx/sqrt(1-TN^2); % = dTNdx * (1-TN^2)^(-1/2)
ddAbductiondx = ddTNdx/sqrt(1-TN^2) + dTNdx * ( -(1/2) * (1-TN^2)^(-3/2) * -2*TN * dTNdx);

return;

% %% Code to prove the equations are right:
% syms PelvisTZ(t) AnkleTZ(t) xHF(t) xKF(t)
% syms l_upper l_lower w_pelvis U
% ss0 = {'PelvisTZ(t)','AnkleTZ(t)','xHF(t)','xKF(t)'};
% sr0 = {'PelvisTZ','AnkleTZ','xHF','xKF'};
% ss1 = {'D(PelvisTZ)(t)','D(AnkleTZ)(t)','D(xHF)(t)','D(xKF)(t)'};
% sr1 = {'dPelvisTZdx','dAnkleTZdx','dxHFdx','dxKFdx'};
% ss2 = {'D(D(PelvisTZ))(t)','D(D(AnkleTZ))(t)','D(D(xHF))(t)','D(D(xKF))(t)'};
% sr2 = {'ddPelvisTZdx','ddAnkleTZdx','ddxHFdx','ddxKFdx'};
% ss = {ss2{:}, ss1{:}, ss0{:}};
% sr = {sr2{:}, sr1{:}, sr0{:}};
% 
% 
% l_leg_projected = cos(xHF) * l_upper + cos(xHF-xKF) * l_lower;
% Ab2 = asin ( (U* (AnkleTZ - PelvisTZ) - (0.5*w_pelvis)) / l_leg_projected);
% dAb2= simple(diff(Ab2,t));
% ddAb2 = diff(dAb2,t);
% 
% Ab3 = subs(Ab2,ss,sr)
% dAb3 = subs(dAb2,ss,sr) % This is the derivative according to matlab
% ddAb3 = subs(ddAb2,ss,sr) % This is the second derivative according to matlab
% 
% % Copy my own equations as syms
% syms PelvisTZ dPelvisTZdx ddPelvisTZdx  ...
%     AnkleTZ dAnkleTZdx ddAnkleTZdx  ...
%     xHF  dxHFdx  ddxHFdx xKF dxKFdx ddxKFdx...
%     w_pelvis l_upper l_lower
% 
% T = U* (AnkleTZ - PelvisTZ) - 0.5*w_pelvis;
% dTdx = U * (dAnkleTZdx - dPelvisTZdx);
% ddTdx = U * (ddAnkleTZdx - ddPelvisTZdx);
% 
% N = cos(xHF) * l_upper + cos(xHF-xKF) * l_lower;
% dNdx = -l_upper * sin(xHF) * dxHFdx - l_lower * sin(xHF-xKF) * (dxHFdx - dxKFdx);
% ddNdx = -l_upper * (cos(xHF) * dxHFdx^2 + sin(xHF) * ddxHFdx) - l_lower * (cos(xHF-xKF)* (dxHFdx-dxKFdx)^2 + sin(xHF-xKF) * (ddxHFdx - ddxKFdx));
% 
% TN = T/N;
% dTNdx = dTdx / N -  (T/(N^2)) * dNdx;
% %ddTNdx = ddTdx/N - dTdx/N^2 * dNdx  - (dTdx/N^2 - 2*T/N^3 * dNdx + (T/N^2)*ddNdx);
% ddTNdx = ddTdx/N - dTdx/N^2*dNdx   -   dTdx/N^2*dNdx + T*dNdx * 2 * N^-3 * dNdx - T/N^2*ddNdx;
% 
% Abduction = asin ( T/N)
% dAbductiondx = simple(dTNdx/sqrt(1-TN^2)) % = dTNdx * (1-TN^2)^(-1/2)
% ddAbductiondx = ddTNdx/sqrt(1-TN^2) + dTNdx * ( -(1/2) * (1-TN^2)^(-3/2) * -2*TN * dTNdx)
% 
% % Check if they're the same; these should all be zero
% er0 = simple(Ab3 - Abduction)
% er1 = simple(dAbductiondx - dAb3)
% er2 = ddAbductiondx - ddAb3
% 
% % er2 is too complex to show analytically. Therefore, let's use random
% %% numbers to show
% U=1;
% PelvisTZ=rand/5; dPelvisTZdx=rand; ddPelvisTZdx=rand;
% AnkleTZ=rand/5; dAnkleTZdx=rand;ddAnkleTZdx=rand;
% xHF=rand/5; dxHFdx=rand; ddxHFdx=rand; xKF=rand/2; dxKFdx=rand; ddxKFdx=rand;
% w_pelvis=abs(rand); l_upper=abs(rand); l_lower=abs(rand);
% (((w_pelvis/2 - U*(AnkleTZ - PelvisTZ))*(ddxHFdx*l_upper*sin(xHF) + dxHFdx^2*l_upper*cos(xHF) + l_lower*sin(xHF - xKF)*(ddxHFdx - ddxKFdx) + l_lower*cos(xHF - xKF)*(dxHFdx - dxKFdx)^2))/(l_upper*cos(xHF) + l_lower*cos(xHF - xKF))^2 + (2*(w_pelvis/2 - U*(AnkleTZ - PelvisTZ))*(dxHFdx*l_upper*sin(xHF) + l_lower*sin(xHF - xKF)*(dxHFdx - dxKFdx))^2)/(l_upper*cos(xHF) + l_lower*cos(xHF - xKF))^3 - (U*(ddAnkleTZdx - ddPelvisTZdx))/(l_upper*cos(xHF) + l_lower*cos(xHF - xKF)) - (2*U*(dAnkleTZdx - dPelvisTZdx)*(dxHFdx*l_upper*sin(xHF) + l_lower*sin(xHF - xKF)*(dxHFdx - dxKFdx)))/(l_upper*cos(xHF) + l_lower*cos(xHF - xKF))^2)/(1 - (w_pelvis/2 - U*(AnkleTZ - PelvisTZ))^2/(l_upper*cos(xHF) + l_lower*cos(xHF - xKF))^2)^(1/2) - ((2*(w_pelvis/2 - U*(AnkleTZ - PelvisTZ))*(dxHFdx*l_upper*sin(xHF) + l_lower*sin(xHF - xKF)*(dxHFdx - dxKFdx))^2)/(l_upper*cos(xHF) + l_lower*cos(xHF - xKF))^3 - (U*(ddAnkleTZdx - ddPelvisTZdx))/(l_upper*cos(xHF) + l_lower*cos(xHF - xKF)) + ((w_pelvis/2 - U*(AnkleTZ - PelvisTZ))*(l_lower*(sin(xHF - xKF)*(ddxHFdx - ddxKFdx) + cos(xHF - xKF)*(dxHFdx - dxKFdx)^2) + l_upper*(cos(xHF)*dxHFdx^2 + ddxHFdx*sin(xHF))))/(l_upper*cos(xHF) + l_lower*cos(xHF - xKF))^2 - (2*U*(dAnkleTZdx - dPelvisTZdx)*(dxHFdx*l_upper*sin(xHF) + l_lower*sin(xHF - xKF)*(dxHFdx - dxKFdx)))/(l_upper*cos(xHF) + l_lower*cos(xHF - xKF))^2)/(1 - (w_pelvis/2 - U*(AnkleTZ - PelvisTZ))^2/(l_upper*cos(xHF) + l_lower*cos(xHF - xKF))^2)^(1/2) - (((2*(w_pelvis/2 - U*(AnkleTZ - PelvisTZ))^2*(dxHFdx*l_upper*sin(xHF) + l_lower*sin(xHF - xKF)*(dxHFdx - dxKFdx)))/(l_upper*cos(xHF) + l_lower*cos(xHF - xKF))^3 - (2*U*(w_pelvis/2 - U*(AnkleTZ - PelvisTZ))*(dAnkleTZdx - dPelvisTZdx))/(l_upper*cos(xHF) + l_lower*cos(xHF - xKF))^2)*((U*(dAnkleTZdx - dPelvisTZdx))/(l_upper*cos(xHF) + l_lower*cos(xHF - xKF)) - ((w_pelvis/2 - U*(AnkleTZ - PelvisTZ))*(dxHFdx*l_upper*sin(xHF) + l_lower*sin(xHF - xKF)*(dxHFdx - dxKFdx)))/(l_upper*cos(xHF) + l_lower*cos(xHF - xKF))^2))/(2*(1 - (w_pelvis/2 - U*(AnkleTZ - PelvisTZ))^2/(l_upper*cos(xHF) + l_lower*cos(xHF - xKF))^2)^(3/2)) - ((w_pelvis/2 - U*(AnkleTZ - PelvisTZ))*((U*(dAnkleTZdx - dPelvisTZdx))/(l_upper*cos(xHF) + l_lower*cos(xHF - xKF)) - ((w_pelvis/2 - U*(AnkleTZ - PelvisTZ))*(dxHFdx*l_upper*sin(xHF) + l_lower*sin(xHF - xKF)*(dxHFdx - dxKFdx)))/(l_upper*cos(xHF) + l_lower*cos(xHF - xKF))^2)^2)/((1 - (w_pelvis/2 - U*(AnkleTZ - PelvisTZ))^2/(l_upper*cos(xHF) + l_lower*cos(xHF - xKF))^2)^(3/2)*(l_upper*cos(xHF) + l_lower*cos(xHF - xKF)))
% % Indeed, it gives 0!

== matlab function LopesDevelopmentLibrary/GaitPhaseDetection/Gait Phase detection/Phase_selection/MATLAB Function ==
  data: left input; y output; right input; belt input; left_x input; right_x input
function y = fcn(left,right,belt,left_x,right_x)
%% If both foot on the ground (1,1), double stance (3)
%% If left foot is in swing, right on ground (4)
%% If right foot is in swing, left on ground -> (2)
%% If belt is still -> (1)
%% else -> (0) (error) 

if belt == 0
    y = 0;
elseif left == 1 && right == 1 && left_x>right_x
    y = 1;
elseif left == 1 && right == 2 
    y = 2;
elseif left == 1 && right == 1 && left_x<right_x
    y = 3;
elseif left == 2 && right == 1
    y = 4;
else 
    y=-1;
end

end

== matlab function LopesDevelopmentLibrary/BlocksForInternalUse/GaitGeneration/SmoothlyRemove2ndKE/SmoothlyRemoveSecondKeyEvent ==
  data: KE_in input; KE_out output; v input
function KE_out = SmoothRemove2ndKeyEvent(KE_in, v)
%#codegen
%
% This block 'smoothly removes' the second key event.
% For v>1.2 m/s, the key event is not removed
% For v<1.0 m/s, the key event is completely removed
% In between, we take a weighed average of when the KE is or is not removed.
% See Technical documentation for details.

% Calculate alpha (i.e., how much of the original key event should we put
% in
v_upper = 1.2; v_lower = 1.0; % m/s
if v>=v_upper
    alpha = 1;
elseif v<=v_lower
    alpha = 0;
else
    alpha = (v-v_lower) / (v_upper-v_lower);
end;

if alpha==1
    % No need for removing the key event
    KE_out = KE_in; 
else
    % Then we need the removed key event; (if alpha==1, we don't)
    phi1 = KE_in(1,1);
    phi2 = KE_in(2,1);
    phi3 = KE_in(3,1);

    % Generate key event K*_2 at the phase of original key event 2
    % For this we do:
    % 1. Get coefficients [c] for the 3rd order polynomial between K1 and K3
    %    y = c3 * x^3 + c2 * x^2 + c1 * x + c0
    %    y' = 3 * c3 * x^2 + 2 * c2 * x + c1
    %    where y, y' and x are known at start and end of the curve, and all cs are unknown.
    %    Rewrite as:
    %    [ y1  ]       [ c3 ]
    %    [ y1' ]       [ c2 ]
    %    [ y3  ] = A * [ c1 ]
    %    [ y3' ]       [ c0 ]
    %
    %    A = [  x1^3,   x1^2,   x1,   1; 
    %         3*x1^2, 2*x1  ,    1,   0;
    %           x3^3,   x3^2,   x3,   1;
    %         3*x3^2, 2*x3  ,    1,   0];
    %   We can shift x to the left by x1, giving new x1=x1-x1=0; x3 = x3-x1
    %   and solve for coefficients vector c.
    x3 = phi3-phi1;
    A = [0, 0, 0, 1; 0, 0, 1,0; x3^3, x3^2, x3, 1; 3*x3^2, 2*x3, 1,0]; 
    y = [KE_in(1,2:3), KE_in(3,2:3)];
    c = A \ y';

    % Now evaluate y2 and y2' (ie, position and velocity of the curve at
    % position phi2) with the same equation as above
    x2 = phi2-phi1;
    A = [x2^3, x2^2, x2, 1; 3*x2^2, 2*x2, 1,0];
    y2 = A * c;

    % Generate new key event as a weighed average of the original K2 and K*.
    KE_out = KE_in;
    KE_out(2,2:3) = (1-alpha) * y2' + alpha * KE_in(2,2:3);
end;

== matlab function LopesDevelopmentLibrary/GaitPhaseDetection/Gait Phase Detection with Wrapper/Phase_selection/MATLAB Function ==
  data: leftWalking input; y output; rightWalking input; leftStop input; rightStop input; switchSignal input; left_x input; right_x input; prev input
function y = fcn(leftWalking,rightWalking,leftStop,rightStop,switchSignal,left_x,right_x,prev)
%% If both foot on the ground (1,1), double stance (3)
%% If left foot is in swing, right on ground (4)
%% If right foot is in swing, left on ground -> (2)
%% If belt is not running, COP detection is used instead of walking detection
%% else -> (-1) (error) 

%% Switching between WalkingDetection/StandingStill detection
if switchSignal == 0    
    left = leftStop; 
    right = rightStop; 
else
    left = leftWalking; 
    right = rightWalking; 
end

%% Setting Phase
if left == 1 && right == 1 && left_x>right_x 
    y_init = 1;
elseif left == 1 && right == 2 
    y_init = 2;
elseif left == 1 && right == 1 && left_x<right_x 
    y_init = 3;
elseif left == 2 && right == 1 
    y_init = 4;
elseif left == 2 && right == 2
    % Flight
    y_init = -2; 
else 
    % Error
    y_init = -1;
end

%% Making sure the sequence (1 2 3 4) is followed in case of walking
if switchSignal == 0
    y = y_init; 
else
    % In case of walking, sequence should always be followed
    % This is checked to throw out false detections
    if y_init == -1 || y_init == -2 || prev == -1 || prev == -2
        % In case of error or flight, just regard the sequence
        y = y_init;
    elseif prev == 0 && (y_init == 2 || y_init == 4);
        y = y_init;
    elseif (((y_init - prev) == 1 || (y_init - prev) == 2)  && y_init ~=1) || (prev == 4 && (y_init == 1 || y_init == 2))
        y = y_init;
    else
        y = prev;
    end
end

end
